simulink model "simulation"  (R2018b)
settings: Solver=FixedStepDiscrete  StartTime=0.0  StopTime=simtime  FixedStep=stepsize  RelTol=1e-3
undefined symbols (not defined in the file): activate_stop, activate_stop_vmax, ay_stop, Bat_param, deltav_ist, DiscIntNeverNeededParam, EG_wunsch, magnitude, mu_road_LF, mu_road_LR, mu_road_RF, mu_road_RR, par_ASR, par_MDT, par_TIR, par_VEH, select_delta_h, select_M_wheel, stepsize, t, temp_betriebsstrategie, temperature_LTrange, track_left, track_right
libraries: Library_ASK x36, simulink x18, dspstat3 x2, Library_Betriebsstrategie x2, vehicle_model x2, pacejka_trans x1
(part 6 of 6)

== system simulation/Vehicle/Betriebsstrategie/Momentenverteilung_und_Schaltstrategie1/Radmomentenaufteilung (Effizienz)/Torque shift damper/Optimierung_damped_AWD ==
  P_achs : Inport
  M_target : Inport  Port=2
  Enable : EnablePort
  Constant : Constant  Value=0.022
  Constant1 : Constant  Value=2
  Memory : Memory  InitialCondition=1
  Memory1 : Memory
  Memory2 : Memory  InitialCondition=1
  Minimierung : MATLAB Function  TreatAsAtomicUnit=on
  Product : Product
  Sign : Signum
  P_opt : Outport
  ind : Outport  Port=2
  wires:
  P_achs/1 -> Minimierung/1(P_achs)
  M_target/1 -> Product/1, Minimierung/4(M_target), Memory2/1
  Constant/1 -> Minimierung/2(difference)
  Memory2/1 -> Product/2
  Constant1/1 -> Minimierung/3(max_oscillation_sec)
  Minimierung/2(ind) -> ind/1, Memory/1
  Memory1/1 -> Minimierung/7(count_prev)
  Memory/1 -> Minimierung/6(ind_prev)
  Minimierung/3(count) -> Memory1/1
  Minimierung/1(P_opt) -> P_opt/1
  Product/1 -> Sign/1
  Sign/1 -> Minimierung/5(change)

== system simulation/Vehicle/Betriebsstrategie/Momentenverteilung_und_Schaltstrategie1/Radmomentenaufteilung (Effizienz)/Torque shift damper/Optimierung_eine_achs ==
  P_achs : Inport
  M_target : Inport  Port=2
  Akt_VA : Inport  Port=3
  Akt_HA : Inport  Port=4
  Enable : EnablePort
  Optimierung : MATLAB Function  TreatAsAtomicUnit=on
  "P_opt " : Outport
  "ind " : Outport  Port=2
  wires:
  Optimierung/1(P_opt) -> "P_opt "/1
  Optimierung/2(ind) -> "ind "/1
  M_target/1 -> Optimierung/2(M_target)
  P_achs/1 -> Optimierung/1(P_achs)
  Akt_VA/1 -> Optimierung/3(VA)
  Akt_HA/1 -> Optimierung/4(HA)

== system simulation/Vehicle/Betriebsstrategie/Momentenverteilung_und_Schaltstrategie1/Radmomentenaufteilung (Effizienz)/Momentenrückführung und Motormomentberechnung/Getriebewirkungsgradberechnung Hinterachse/Falls radnahe Maschine an HA1 ==
  M_HA : Inport
  Constant1 : Constant  Value=par_MDT.AUS.akt.az_HA
  Gain : Gain  Gain=0.5
  Switch : Switch  Criteria=u2 > Threshold
  M_HA_mot : Outport
  wires:
  Constant1/1 -> Switch/2
  M_HA/1 -> Switch/1, Gain/1
  Gain/1 -> Switch/3
  Switch/1 -> M_HA_mot/1

== system simulation/Vehicle/Betriebsstrategie/Momentenverteilung_und_Schaltstrategie1/Radmomentenaufteilung (Effizienz)/Momentenrückführung und Motormomentberechnung/Getriebewirkungsgradberechnung Hinterachse/Falls radnahe Maschine an HA2 ==
  M_HA : Inport
  Constant1 : Constant  Value=par_MDT.AUS.akt.az_HA
  Gain : Gain  Gain=2
  Switch : Switch  Criteria=u2 > Threshold
  M_HA_mot : Outport
  wires:
  Constant1/1 -> Switch/2
  M_HA/1 -> Switch/1, Gain/1
  Gain/1 -> Switch/3
  Switch/1 -> M_HA_mot/1

== system simulation/Vehicle/Betriebsstrategie/Momentenverteilung_und_Schaltstrategie1/Radmomentenaufteilung (Effizienz)/Momentenrückführung und Motormomentberechnung/Getriebewirkungsgradberechnung Vorderachse/Falls radnahe Maschine an VA ==
  M_VA : Inport
  Constant1 : Constant  Value=par_MDT.AUS.akt.az_VA
  Gain : Gain  Gain=0.5
  Switch : Switch  Criteria=u2 > Threshold
  M_VA_mot : Outport
  wires:
  Constant1/1 -> Switch/2
  M_VA/1 -> Switch/1, Gain/1
  Gain/1 -> Switch/3
  Switch/1 -> M_VA_mot/1

== system simulation/Vehicle/Betriebsstrategie/Momentenverteilung_und_Schaltstrategie1/Radmomentenaufteilung (Effizienz)/Momentenrückführung und Motormomentberechnung/Getriebewirkungsgradberechnung Vorderachse/Falls radnahe Maschine an VA1 ==
  M_VA : Inport
  Constant1 : Constant  Value=par_MDT.AUS.akt.az_VA
  Gain : Gain  Gain=2
  Switch : Switch  Criteria=u2 > Threshold
  M_VA_mot : Outport
  wires:
  Constant1/1 -> Switch/2
  M_VA/1 -> Switch/1, Gain/1
  Gain/1 -> Switch/3
  Switch/1 -> M_VA_mot/1

== matlab function simulation/Driver/Splines/Kennwerte ==
  data: psi_old input; psi_spline output; time input; a1 input; a0 input; v2 input; v1 input; v0 input; p3 input; p2 input; p1 input; p0 input; psi_real input; spl_a_glob output; spl_v_glob output; spl_p_glob output; spl_a_veh output; spl_v_veh output; p_err_long output; p_ist input; p_err_lat output
function [ psi_spline, spl_a_glob, spl_v_glob, spl_p_glob, spl_a_veh, spl_v_veh, p_err_long, p_err_lat]   = Kennwerte(psi_old, time, a1, a0, v2, v1, v0, p3, p2, p1, p0, psi_real, p_ist) 
%Splinekoeffizienten im Abstand von 0.01 s, deshalb wird Zeit mit 100 
%mulitpliziert,um alle 0.01 s auf nächsten Spline-Koeffizienten zuzugreifen
time = time * 100;
%t wird angelegt, damit extrapoliert werden kann, wenn die Zeit über die
%vorgesehene Zeit im Struct hinausreicht
t = time;
if time > length(a0)-2
    time = length(a0)-2;
end

si = int16(floor(time)+1); %Spline Index, Auswahl des Richtigen Splines 
ov = t-floor(time); %Overshoot, Zeit nach dem Beginn des Spline

%%Berechnung der Beschleunigung a, Geschwindigkeit v und Position p in globalen Koordianten
spl_a_glob =  a1(:,si).*(ov)   +a0(:,si);
spl_v_glob =  v2(:,si).*(ov).^2+v1(:,si).*(ov)   +v0(:,si);
spl_p_glob =  p3(:,si).*(ov).^3+p2(:,si).*(ov).^2+p1(:,si).*(ov)+p0(:,si);

%%Verhindert Springen des Gierwinkels bei niedrigen Geschwindigkeiten
if spl_v_glob(1) < 1e-5 && spl_v_glob(2) < 1e-5
     psi_spline = psi_old;
else
     psi_spline = atan2(spl_v_glob(2),spl_v_glob(1)); %Gierwinkel soll
end

psi = psi_spline; %Optional kann die tatsächliche Fahrzeugausrichtung verwendet werden
tm  = [cos(psi) sin(psi); -sin(psi) cos(psi)]; %Transformations-Matrix

spl_a_veh = tm * spl_a_glob; %Beschleunigung soll in Fahrzeugsollkoordinaten
spl_v_veh = tm * spl_v_glob; %Geschwindigkeit soll in Fahrzeugsollkoordinaten


p_veh = tm * (p_ist - spl_p_glob);
p_err_long = p_veh(1); %Lateraler Fehler in Fahrzeugsollkoordinaten
p_err_lat = p_veh(2); %Longitudinaler in Fahrzeugsollkoordinaten

end

== matlab function simulation/Vehicle/Antriebsstrang und Radmomentenverteilung/Batterie/MATLAB Function2 ==
  data: u input; y output
function y = fcn(u)
%Transponieren der Leistung -> für das Batteriemodell

y=reshape(u,[1,1,[]]);


end

== matlab function simulation/Vehicle/Betriebsstrategie/Momentenverteilung_und_Schaltstrategie1/Radmomentenaufteilung (Effizienz)/Momentenrückführung und Motormomentberechnung/Getriebewirkungsgradberechnung Vorderachse/MATLAB Function ==
  data: M_out input; M_in output; M_max input
function M_in = fcn(M_out, M_max)
M_in = 3/680 *((sqrt(M_max) * sqrt(27*M_max + 27200*M_out))/sqrt(3) - 3 * M_max)

== matlab function simulation/Driver/driver lateral/Pure Pursuit/MATLAB Function ==
  data: oldtime input; lad input; time input; v2 input; v1 input; v0 input; p3 input; p2 input; p1 input; p0 input; p_ist input; time_out output; dt output; err output; cp output
function [time_out, dt, err, cp]    = Carott(oldtime, lad, time,v2, v1, v0, p3, p2, p1, p0, p_ist)

t = oldtime; %Übernahme der Zeit aus letztem Zeitschritt

%Verhindert einen Zeitindex außerhalb der Matrixgröße
if oldtime > length(p0)-2
    oldtime = length(p0)-2;
elseif oldtime < 0
    oldtime = 0
end


si = int16(floor(oldtime)+1); %Spline Index, Auswahl des Richtigen Splines 
ov = t-floor(oldtime); %Overshoot, Zeit nach dem Beginn des Spline
cp =  p3(:,si).*(ov).^3+p2(:,si).*(ov).^2+p1(:,si).*(ov)+p0(:,si); %Berechnung des CP bei prognostizierter Zeit 


dist = norm(cp-p_ist); %Abstand Carrot-Point zum Fahrzeug
err = abs(1-dist/lad) %Normierung des Fehlers auf LAD
dt = 0; %Zeitdifferenz wird genullt

    v =  norm(v2(:,si).*(ov).^2+v1(:,si).*(ov)  +v0(:,si)); %FZG-Geschwindigkeit wird berechnet
    if v < 0.3 %Mindestgeschwindigkeit um CP bei Stillstand zu ermitteln 
        v = 0.3
    end
    dt = dt + (lad-dist)/v*100; %Zeitdifferenz wird aus Abstandsfehler und Geschwindigkeit ermittelt
    newtime = oldtime + dt; %Neuer Zeitpunkt, auf dem sich CP befindet, wird prognostiziert
    t = newtime; %Übernahme der prognostizierten Zeit
    
    %Verhindert einen Zeitindex außerhalb der Matrixgröße
    if newtime > length(p0)-2
        newtime = length(p0)-2;
    elseif newtime < 0
        newtime = 0
    end
    
    si = int16(floor(newtime)+1); %Spline Index, Auswahl des Richtigen Splines 
    ov = t-floor(newtime); %Overshoot, Zeit nach dem Beginn des Spline
    cp =  p3(:,si).*(ov).^3+p2(:,si).*(ov).^2+p1(:,si).*(ov)+p0(:,si); %Berechnung des CP bei neuer prognostizierter Zeit 
    dist = norm(cp-p_ist); %Abstand Carrot-Point zum Fahrzeug
    err = abs(1-dist/lad) %Normierung des Fehlers auf LAD

time_out = oldtime + dt; %Neuer Zeitpunkt, auf dem sich CP befindet, wird prognostiziert
end

== matlab function simulation/Vehicle/Betriebsstrategie/Momentenverteilung_und_Schaltstrategie1/Radmomentenaufteilung (Effizienz)/Momentenrückführung und Motormomentberechnung/Getriebewirkungsgradberechnung Hinterachse/MATLAB Function1 ==
  data: M_out input; M_in output; M_max input
function M_in = fcn(M_out, M_max)
M_in = 3/680 *((sqrt(M_max) * sqrt(27*M_max + 27200*M_out))/sqrt(3) - 3 * M_max)

== matlab function simulation/Vehicle/Antriebsstrang und Radmomentenverteilung/Batterie/MATLAB Function3 ==
  data: u input; y output
function y = fcn(u)
%Zusammenfassung der Verluste der LE auf eine Vektorspalte -> für das
%Batteriemodell


y=reshape(u,[[],1,1]);



end

== matlab function simulation/Vehicle/Antriebsstrang und Radmomentenverteilung/MATLAB Function2 ==
  data: u input; RIX output
function RIX = fcn(u)
%RIX = 1 für Antrieb an mindestens einem Rad, sonst -1
s = (sign(u) == 1);
if all(s) == 0
    RIX = -1;
else
    RIX = 1;
end
end

== matlab function simulation/Vehicle/Antriebsstrang und Radmomentenverteilung/MATLAB Function3 ==
  data: u input; RIX output
function RIX = fcn(u)
%RIX = 1 für Antrieb an mindestens einem Rad, sonst -1
s = (sign(u) == 1);
if all(s) == 0
    RIX = -1;
else
    RIX = 1;
end
end

== matlab function simulation/Vehicle/Betriebsstrategie/Momentenverteilung_und_Schaltstrategie1/Limitierungen gesamt (mit MVS Limits)/Aktuatoren und Delta TV/TV Moment pro Achse ==
  data: L1 input; Delta_T_f output; L2 input; L3 input; L4 input; L5 input; a_f input; a_r input; Delta_T_r output
function [Delta_T_f, Delta_T_r]  = fcn(L1, L2, L3, L4, L5, a_f, a_r)

%% Initialisierung
Delta_T_f=0;
Delta_T_r=0;

%% Zuweisung der maximalen TV Momente anhand der Antriebsstrangtopologie
if a_f == 3
    Delta_T_f=L5;
elseif a_f == 4
    Delta_T_f=L1;
elseif a_f == 5
    Delta_T_f=L2;
end

if a_r == 3
    Delta_T_r=L5;
elseif a_r == 4
    Delta_T_r=L1;
elseif a_r == 5
    Delta_T_r=L2;
end

%% Nomenklatur der Aktuatoren a_r und a_f
    % 1 = nur Elektromaschinen an der Achse
    % 2 = Offenes Differential an der Achse
    % 3 = Limited Slip Differential an der Achse
    % 4 = Elektrisches Überlagerungsgetriebe an der Achse
    % 5 = Mechanisches Überlagerungsgetriebe an der Achse

== matlab function simulation/Vehicle/Antriebsstrang und Radmomentenverteilung/MATLAB Function4 ==
  data: u input; RIX output
function RIX = fcn(u)
%RIX = 1 für Antrieb an mindestens einem Rad, sonst -1
s = (sign(u) == 1);
if all(s) == 0
    RIX = -1;
else
    RIX = 1;
end
end

== matlab function simulation/Vehicle/Antriebsstrang und Radmomentenverteilung/MATLAB Function5 ==
  data: u input; RIX output
function RIX = fcn(u)
%RIX = 1 für Antrieb an mindestens einem Rad, sonst -1
s = (sign(u) == 1);
if all(s) == 0
    RIX = -1;
else
    RIX = 1;
end
end

== matlab function simulation/Vehicle/Betriebsstrategie/Momentenverteilung_und_Schaltstrategie1/Limitierungen gesamt (mit MVS Limits)/Aktuatoren und Delta TV/Zuweisung Aktuatoren ==
  data: A1 input; A2 input; A3 input; A4 input; A5 input; a_f output; a_r output; A6 input; A7 input; A8 input; A9 input; A10 input
function [a_f, a_r]  = fcn(A1, A2, A3, A4, A5, A6, A7, A8, A9, A10)

%% Initialisierung
a_f=1;
a_r=1;

%% Zuweisung der Aktuatoren
% vorne
if A1 == 1
    a_f = 2;
elseif A2 == 1
    a_f = 3;
elseif A3 == 1
    a_f = 5;
elseif A4 == 1
    a_f = 4;
elseif A5 == 1
    a_f = 1;
end

% hinten
if A6 == 1
    a_r = 2;
elseif A7 == 1
    a_r = 3;
elseif A8 == 1
    a_r = 5;
elseif A9 == 1
    a_r = 4;
elseif A10 == 1
    a_r = 1;
end

%% Nomenklatur der Aktuatoren a_r und a_f
    % 1 = nur Elektromaschinen an der Achse
    % 2 = Offenes Differential an der Achse
    % 3 = Limited Slip Differential an der Achse
    % 4 = Elektrisches Überlagerungsgetriebe an der Achse
    % 5 = Mechanisches Überlagerungsgetriebe an der Achse

== matlab function simulation/Vehicle/Antriebsstrang und Radmomentenverteilung/MATLAB Function ==
  data: u input; RIX output
function RIX = fcn(u)
%RIX = 1 für Antrieb an mindestens einem Rad, sonst -1
s = (sign(u) == 1);
if all(s) == 0
    RIX = -1;
else
    RIX = 1;
end
end

== matlab function simulation/Vehicle/Antriebsstrang und Radmomentenverteilung/MATLAB Function1 ==
  data: u input; RIX output
function RIX = fcn(u)
%RIX = 1 für Antrieb an mindestens einem Rad, sonst -1
s = (sign(u) == 1);
if all(s) == 0
    RIX = -1;
else
    RIX = 1;
end
end

== matlab function simulation/Vehicle/Betriebsstrategie/Momentenverteilung_und_Schaltstrategie1/Limitierungen gesamt (mit MVS Limits)/Limits Zusammenführung ==
  data: FxlimRF input; FxlimLF input; FxlimRR input; Fx_LF_ub output; Fx_LF_lb output; Fx_RF_ub output; Fx_RF_lb output; Fx_LR_ub output; Fx_LR_lb output; Fx_RR_ub output; Fx_RR_lb output; FxlimLR input; M_RF_ub input; M_RF_lb input; M_LF_ub input; M_LF_lb input; M_RR_ub input; M_RR_lb input; M_LR_ub input; M_LR_lb input; M_F_lb input; M_F_ub input; M_R_lb input; M_R_ub input; DELTA_T_f input; DELTA_T_r input; a_f input; a_r input; r input
function [Fx_LF_ub, Fx_LF_lb, Fx_RF_ub, Fx_RF_lb, Fx_LR_ub, Fx_LR_lb, Fx_RR_ub, Fx_RR_lb] = fcn(FxlimRF, FxlimLF, FxlimRR, FxlimLR, M_RF_ub, M_RF_lb, M_LF_ub, M_LF_lb, M_RR_ub, M_RR_lb, M_LR_ub, M_LR_lb, M_F_lb, M_F_ub, M_R_lb, M_R_ub,DELTA_T_f, DELTA_T_r,a_f, a_r, r)

% Reifenverhalten beim Antreiben und Bremsen gleich
Fx_LF_ub = FxlimLF;
Fx_RF_ub = FxlimRF;
Fx_LF_lb = (-1*FxlimLF);
Fx_RF_lb = (-1*FxlimRF);

Fx_LR_ub = FxlimLR;
Fx_RR_ub = FxlimRR;
Fx_LR_lb = (-1*FxlimLR);
Fx_RR_lb = (-1*FxlimRR);

% Notwendig, da die Rekuperationskennfelder aus dem Pesche Tool positive
% Momente ausgeben
M_RF_lb=(-1)*M_RF_lb;
M_LF_lb=(-1)*M_LF_lb;
M_RR_lb=(-1)*M_RR_lb;
M_LR_lb=(-1)*M_LR_lb;
M_F_lb=(-1)*M_F_lb;
M_R_lb=(-1)*M_R_lb;
    
%% Nomenklatur der Aktuatoren a_r und a_f
    % 1 = nur Elektromaschinen an der Achse
    % 2 = Offenes Differential an der Achse
    % 3 = Limited Slip Differential an der Achse
    % 4 = Elektrisches Überlagerungsgetriebe an der Achse
    % 5 = Mechanisches Überlagerungsgetriebe an der Achse
 
    
%% Nur Elektromotoren: Limit ist Minimum/Maximum aus Reifenlimit und Limit der EM
if a_f == 1
    Fx_LF_ub = min(FxlimLF,(M_LF_ub/r));
    Fx_RF_ub = min(FxlimRF,(M_RF_ub/r));
    Fx_LF_lb = max((-1*FxlimLF),(M_LF_lb/r));
    Fx_RF_lb = max((-1*FxlimRF),(M_RF_lb/r));
end

if a_r == 1
    Fx_LR_ub = min(FxlimLR,(M_LR_ub/r));
    Fx_RR_ub = min(FxlimRR,(M_RR_ub/r));
    Fx_LR_lb = max((-1*FxlimLR),(M_LR_lb/r));
    Fx_RR_lb = max((-1*FxlimRR),(M_RR_lb/r));
end

%% Offenes Differential: Limit ist Minimum/Maximum aus Reifenlimit und genau der Hälfte des max. Moments der achszentralen EM
if a_f == 2
    Fx_LF_ub = min(FxlimLF,(0.5*M_F_ub/r));
    Fx_RF_ub = min(FxlimRF,(0.5*M_F_ub/r));
    Fx_LF_lb = max((-1*FxlimLF),(0.5*M_F_lb/r));
    Fx_RF_lb = max((-1*FxlimRF),(0.5*M_F_lb/r));
end

if a_r == 2
    Fx_LR_ub = min(FxlimLR,(0.5*M_R_ub/r));
    Fx_RR_ub = min(FxlimRR,(0.5*M_R_ub/r));
    Fx_LR_lb = max((-1*FxlimLR),(0.5*M_R_lb/r));
    Fx_RR_lb = max((-1*FxlimRR),(0.5*M_R_lb/r));
end

%% Limited Slip Differential %% Elektrisches Überlagerungsgetriebe %% Mechanisches Überlagerungsgetriebe:
if a_f >= 3 
    Fx_LF_ub = min(FxlimLF,(0.5*M_F_ub/r + 0.5*DELTA_T_f/r));
    Fx_RF_ub = min(FxlimRF,(0.5*M_F_ub/r + 0.5*DELTA_T_f/r));
    Fx_LF_lb = max((-1*FxlimLF),(0.5*M_F_lb/r - 0.5*DELTA_T_f/r));
    Fx_RF_lb = max((-1*FxlimRF),(0.5*M_F_lb/r - 0.5*DELTA_T_f/r));
end

if a_r >= 3
    Fx_LR_ub = min(FxlimLR,(0.5*M_R_ub/r + 0.5*DELTA_T_r/r));
    Fx_RR_ub = min(FxlimRR,(0.5*M_R_ub/r + 0.5*DELTA_T_r/r));
    Fx_LR_lb = max((-1*FxlimLR),(0.5*M_R_lb/r - 0.5*DELTA_T_r/r));
    Fx_RR_lb = max((-1*FxlimRR),(0.5*M_R_lb/r - 0.5*DELTA_T_r/r));
end


%% kein Antrieb an der achse
if a_f >= 4
    Fx_LF_ub = min(FxlimLF,(0.5*M_F_ub/r + 0.5*DELTA_T_f/r));
    Fx_RF_ub = min(FxlimRF,(0.5*M_F_ub/r + 0.5*DELTA_T_f/r));
    Fx_LF_lb = max((-1*FxlimLF),(0.5*M_F_lb/r - 0.5*DELTA_T_f/r));
    Fx_RF_lb = max((-1*FxlimRF),(0.5*M_F_lb/r - 0.5*DELTA_T_f/r));
end

if a_r >= 4
    Fx_LR_ub = min(FxlimLR,(0.5*M_R_ub/r + 0.5*DELTA_T_r/r));
    Fx_RR_ub = min(FxlimRR,(0.5*M_R_ub/r + 0.5*DELTA_T_r/r));
    Fx_LR_lb = max((-1*FxlimLR),(0.5*M_R_lb/r - 0.5*DELTA_T_r/r));
    Fx_RR_lb = max((-1*FxlimRR),(0.5*M_R_lb/r - 0.5*DELTA_T_r/r));
end

%% Torque Splitter
if a_f == 5
    Fx_LF_ub = min(FxlimLF,(M_F_ub/r));
    Fx_RF_ub = min(FxlimRF,(M_F_ub/r));
    Fx_LF_lb = max((-1*FxlimLF),(M_F_lb/r - DELTA_T_f/r));
    Fx_RF_lb = max((-1*FxlimRF),(M_F_lb/r - DELTA_T_f/r));
end

if a_r == 5
    Fx_LR_ub = min(FxlimLR,(M_R_ub/r));
    Fx_RR_ub = min(FxlimRR,(M_R_ub/r));
    Fx_LR_lb = max((-1*FxlimLR),(M_R_lb/r - DELTA_T_r/r));
    Fx_RR_lb = max((-1*FxlimRR),(M_R_lb/r - DELTA_T_r/r));
end

== matlab function simulation/Vehicle/Betriebsstrategie/Momentenverteilung_und_Schaltstrategie1/Radmomentenaufteilung (Effizienz)/Torque shift damper/Optimierung_eine_achs/Optimierung ==
  data: P_achs input; P_opt output; ind output; M_target input; VA input; HA input
function [P_opt, ind]= fcn(P_achs, M_target, VA, HA)

[n_gears, leng] = size(P_achs);

if HA == 1
    if M_target>0
        [P_opt, ind] = min(P_achs(:,1));
    else
        [P_opt, ind] = max(P_achs(:,1));
    end
else
    if M_target>0
        [P_opt, ind] = min(P_achs(:,leng));
    else
        [P_opt, ind] = max(P_achs(:,leng));
    end
    ind = ind+100*n_gears
end

end

== matlab function simulation/Vehicle/Betriebsstrategie/Momentenverteilung_und_Schaltstrategie1/Radmomentenaufteilung (Standardfahrmanöver)/Limits berücksichtigen ==
  data: Fx_RF output; Fx_LF output; Fx_RR output; Fx_LF_ub input; Fx_LF_lb input; Fx_RF_ub input; Fx_RF_lb input; Fx_LR_ub input; Fx_LR_lb input; Fx_RR_ub input; Fx_RR_lb input; a_f input; a_r input; Fx_LR output; X_FL input; X_FR input; X_RL input; X_RR input
function [Fx_RF, Fx_LF, Fx_RR, Fx_LR] = fcn(Fx_LF_ub, Fx_LF_lb, Fx_RF_ub, Fx_RF_lb, Fx_LR_ub, Fx_LR_lb, Fx_RR_ub, Fx_RR_lb,a_f, a_r, X_FL, X_FR, X_RL, X_RR)

%% Initialisierung
Fx_RF = X_FR;
Fx_LF = X_FL;
Fx_RR = X_RR;
Fx_LR = X_RL;
    
%% Nomenklatur der Aktuatoren a_r und a_f
    % 1 = nur Elektromaschinen an der Achse
    % 2 = Offenes Differential an der Achse
    % 3 = Limited Slip Differential an der Achse
    % 4 = Elektrisches Überlagerungsgetriebe an der Achse
    % 5 = Mechanisches Überlagerungsgetriebe an der Achse
 
%% Algorithmus

    F_f= Fx_RF+Fx_LF;
    F_r= Fx_RR+Fx_LR;
  
  % Nur Elektromotoren:
  % Es werden radindividuell die Grenzen eingehalten. Die Differenzkräfte
  % werden zur späteren Verwendung gespeichert.
if a_f ==1
    if Fx_LF > Fx_LF_ub
        dFx_LF = Fx_LF-Fx_LF_ub;
        Fx_LF = Fx_LF_ub;
    end
    if Fx_RF > Fx_RF_ub
        dFx_RF = Fx_RF-Fx_RF_ub;
        Fx_RF = Fx_RF_ub;
    end
    if Fx_LF < Fx_LF_lb
        dFx_LF = Fx_LF-Fx_LF_lb;
        Fx_LF = Fx_LF_lb;
    end
    if Fx_RF < Fx_RF_lb
        dFx_RF = Fx_RF-Fx_RF_lb;
        Fx_RF = Fx_RF_lb;
    end
end

if a_r ==1
    if Fx_LR > Fx_LR_ub
        dFx_LR = Fx_LR-Fx_LR_ub;
        Fx_LR = Fx_LR_ub;
    end
    if Fx_RR > Fx_RR_ub
        dFx_RR = Fx_RR-Fx_RR_ub;
        Fx_RR = Fx_RR_ub;
    end
    if Fx_LR < Fx_LR_lb
        dFx_LR = Fx_LR-Fx_LR_lb;
        Fx_LR = Fx_LR_lb;
    end
    if Fx_RR < Fx_RR_lb
        dFx_RR = Fx_RR-Fx_RR_lb;
        Fx_RR = Fx_RR_lb;
    end
end

  % Offenes Differential:
  % ALSO keine TV Funktion der Achse.
  % Jedes Rad erhält die Hälfte der Gesamtachskraft.
  % Anschließend wird diese Kraft auf das Minimum der einzelnen Limits
  % gedeckelt.

  %Berücksichtigung bereits in Lagrange-Block
  
if a_f ==2
    Fx_LF = F_f/2;
    Fx_RF = F_f/2;
    if Fx_LF > Fx_LF_ub || Fx_RF > Fx_RF_ub
        Fx_LF = min(Fx_LF_ub,Fx_RF_ub);
        Fx_RF = Fx_LF;
    end
    if Fx_LF < Fx_LF_lb || Fx_RF < Fx_RF_lb
        Fx_LF = max(Fx_LF_lb,Fx_RF_lb);
        Fx_RF = Fx_LF;
    end
end

if a_r ==2
    Fx_LR = F_r/2;
    Fx_RR = F_r/2;
    if Fx_LR > Fx_LR_ub || Fx_RR > Fx_RR_ub
        Fx_LR = min(Fx_LR_ub,Fx_RR_ub);
        Fx_RR = Fx_LR;
    end
    if Fx_LR < Fx_LR_lb || Fx_RR < Fx_RR_lb
        Fx_LR = max(Fx_LR_lb,Fx_RR_lb);
        Fx_RR = Fx_LR;
    end
end
    
%% Limited Slip Differential %% Elektrisches Überlagerungsgetriebe %% Mechanisches Überlagerungsgetriebe
if a_f >=3
    if Fx_LF > Fx_LF_ub
        dFx_LF = Fx_LF-Fx_LF_ub;
        Fx_LF = Fx_LF_ub;
    end
    if Fx_RF > Fx_RF_ub
        dFx_RF = Fx_RF-Fx_RF_ub;
        Fx_RF = Fx_RF_ub;
    end
    if Fx_LF < Fx_LF_lb
        dFx_LF = Fx_LF-Fx_LF_lb;
        Fx_LF = Fx_LF_lb;
    end
    if Fx_RF < Fx_RF_lb
        dFx_RF = Fx_RF-Fx_RF_lb;
        Fx_RF = Fx_RF_lb;
    end
end

if a_r >=3
    if Fx_LR > Fx_LR_ub
        dFx_LR = Fx_LR-Fx_LR_ub;
        Fx_LR = Fx_LR_ub;
    end
    if Fx_RR > Fx_RR_ub
        dFx_RR = Fx_RR-Fx_RR_ub;
        Fx_RR = Fx_RR_ub;
    end
    if Fx_LR < Fx_LR_lb
        dFx_LR = Fx_LR-Fx_LR_lb;
        Fx_LR = Fx_LR_lb;
    end
    if Fx_RR < Fx_RR_lb
        dFx_RR = Fx_RR-Fx_RR_lb;
        Fx_RR = Fx_RR_lb;
    end
end
    
%% Korrektur des TV Moments %% Korrektur des Gesamtmoments

== matlab function simulation/Vehicle/Betriebsstrategie/Momentenverteilung_und_Schaltstrategie1/Radmomentenaufteilung (Effizienz)/Torque shift damper/Optimierung_damped_AWD/Minimierung ==
  data: P_achs input; P_opt output; ind output; count output; difference input; max_oscillation_sec input; M_target input; change input; ind_prev input; count_prev input
function [P_opt, ind, count]= fcn(P_achs, difference, max_oscillation_sec, M_target, change, ind_prev, count_prev)

[leng, x] = size(P_achs);
if M_target>0
    [P_opt, ind] = min(P_achs(:));

    if (P_opt < (1-difference)*P_achs(ind_prev) && count_prev > (leng*2000/max_oscillation_sec)) || change == -1 || isnan(P_achs(ind_prev)) == 1
        count = 0
    else
        ind = ind_prev;
        P_opt = P_achs(ind_prev);
        count = count_prev+1;
    end

else
    [P_opt, ind] = max(P_achs(:));
    
    if (P_opt > (1+difference)*P_achs(ind_prev) && count_prev > (leng*2000/max_oscillation_sec)) || change == -1 || isnan(P_achs(ind_prev)) == 1
        count = 0
    else
        ind = ind_prev;
        P_opt = P_achs(ind_prev);
        count = count_prev+1;
    end
end

end

== matlab function simulation/Vehicle/Betriebsstrategie/Momentenverteilung_und_Schaltstrategie1/Radmomentenaufteilung (Standardfahrmanöver)/Optimierung mit Lagrange Multiplikator Methode ==
  data: a_f input; a_r input; X_req input; Z_FL input; Z_FR input; Z_RL input; Z_RR input; Mz input; tF input; tR input; lf input; lr input; delta input; X_FL output; X_FR output; X_RL output; X_RR output; X_FL1 input; X_FR1 input; X_RL1 input; X_RR1 input
function [X_FL, X_FR, X_RL, X_RR] = fcn(a_f, a_r, X_req, Z_FL, Z_FR, Z_RL, Z_RR, Mz, tF, tR, lf, lr, delta, X_FL1, X_FR1, X_RL1, X_RR1)

%% Auswahl der Antriebsstrantopologie
a=1;
b=1;

if a_f ==2
    a=0;
end
if a_r ==2
    b=0;
end

if a_f ==2 && a_r==2
    a=1;
    b=1;
end

% TV vorne und hinten möglich a=1 und b=1
% TV nur vorne möglich a=1
% TV nur hinten möglich b=1
% kein TV möglich a=1 und b=1 und anschließend gleichmäßig aufteilen

%% Matrix für die Randbedingungen ( Gesamtmoment und TV Moment)
% B0 = [cos(delta) cos(delta) 1 1; a*((-tF/2)*cos(delta)+lf*sin(delta)) a*((tF/2)*cos(delta)+lf*sin(delta)) b*(-tR/2) b*(tR/2)];
% Die Berücksichtigung der Lenkwinkel für die Formel des Gesamtmoments und des Giermomenmts ist exakt, wird
% aber hier erstmal auskommentiert, da ein instabiler Fahrerregler
% vorliegt. Sobald der Fahrerregler komplett stabil ist, kann die obere
% Matrix für B0 verwendet werden.
B0 = [1 1 1 1; a*(-tF/2) a*(tF/2) b*(-tR/2) b*(tR/2)];
y0 = [X_req; Mz];

%% Algorithmus
    %% Initialbedingungen
i=0;    
B=B0;
y=y0;
     
    %% Verhindern abgehobener Räder
if Z_FL < 1
    Z_FL = 1;
    x_FL_max = 0;
end

if Z_FR < 1
    Z_FR = 1;
    x_FR_max = 0;
end

if Z_RL < 1
    Z_RL = 1;
    x_RL_max = 0;
end

if Z_RR < 1
    Z_RR = 1;
    x_RR_max = 0;
end

%% Matrizen für die Mimimierung
W1 = [1/Z_FL 0 0 0; 0 1/Z_FR 0 0; 0 0 1/Z_RL 0; 0 0 0 1/Z_RR];
W2 = 0.01 * eye(4);
%Wquad = W1^2 + W2^2;
Wquad = W1 + W2^2;
X_alt = [X_FL1; X_FR1; X_RL1; X_RR1];

%% Minimierungsargument
% min ||W1*x||^2 + ||W2*(x-x0)||^2
%   ||W1*x||^2 + ||W2*(x-x0)||^2 = xt*W1^2*x + (x-x0)t*W2^2*(x-x0)
%   = xt*(W1^2+W2^2)*x - 2*x*W2^2*x0 + x0*W2^2*x0
%   = xt*W^2*x - 2*x*W2^2*x0 + Konstante
%   mit W^2 = W1^2 + W2^2

%% Berechnung von Xij
G = (Wquad^(-1))*(B')*(B*(Wquad^(-1))*(B'))^(-1);
X = G*y + (eye(4)-G*B)*(Wquad^(-1))*(W2^2)*X_alt;


%% Ausgabewerte berechnen
X_FL = X(1);
X_FR = X(2);
X_RL = X(3);
X_RR = X(4);

%% Limits berücksichtigen
if a==0
    X_F = X_FL + X_FR;
    X_FL = X_F/2;
    X_FR = X_F/2;
end

if b==0
    X_R = X_RL + X_RR;
    X_RL = X_R/2;
    X_RR = X_R/2;
end

if a_f ==2 && a_r==2
    X_F = X_FL + X_FR;
    X_FL = X_F/2;
    X_FR = X_F/2;
    X_R = X_RL + X_RR;
    X_RL = X_R/2;
    X_RR = X_R/2;
end

== matlab function simulation/Vehicle/Betriebsstrategie/Momentenverteilung_und_Schaltstrategie1/Radmomentenaufteilung (Standardfahrmanöver)/Schaltstrategie/Getriebe- wirkungs- grade ==
  data: eta_LF output; eta_RF output; eta_LR output; eta_RR output; eta_F output; eta_R output; idx_LF input; idx_RF input; idx_LR input; idx_RR input; idx_F input; idx_R input; ETA_F input; ETA_R input
function [eta_LF, eta_RF, eta_LR, eta_RR, eta_F, eta_R] = fcn(idx_LF, idx_RF, idx_LR, idx_RR, idx_F, idx_R, ETA_F, ETA_R)

eta_LF=ETA_F(idx_LF);
eta_RF=ETA_F(idx_RF);
eta_LR=ETA_R(idx_LR);
eta_RR=ETA_R(idx_RR);
eta_F=ETA_F(idx_F);
eta_R=ETA_R(idx_R);

% Der Wirkungsgrad des Getriebes im eingelegten Gang wird weitergegeben.
% Frederik benötigt diesen im Antriebsstrangmodell.

== matlab function simulation/Vehicle/Betriebsstrategie/Momentenverteilung_und_Schaltstrategie1/Radmomentenaufteilung (Standardfahrmanöver)/Schaltstrategie/Radmoment zu Motormoment ==
  data: i_LF input; i_RF input; i_LR input; i_RR input; i_F input; i_R input; M_LF input; m_LF output; M_RF input; M_LR input; M_RR input; m_RF output; m_LR output; m_RR output; m_F output; m_R output
function [m_LF, m_RF, m_LR, m_RR, m_F, m_R] = fcn(i_LF, i_RF, i_LR, i_RR, i_F, i_R, M_LF, M_RF, M_LR, M_RR)

%% Motormoment Achszentraler Aufbau
m_F=(M_LF+M_RF)/i_F;
m_R=(M_LR+M_RR)/i_R;

%% Motormoment Radindividueller Aufbau
m_LF=M_LF/i_LF;
m_RF=M_RF/i_RF;
m_LR=M_LR/i_LR;
m_RR=M_RR/i_RR;

== matlab function simulation/Vehicle/Betriebsstrategie/Momentenverteilung_und_Schaltstrategie1/Radmomentenaufteilung (Standardfahrmanöver)/Schaltstrategie/Schaltlogik ==
  data: delta_n_LF input; delta_n_RF input; delta_n_LR input; delta_n_RR input; delta_n_F input; delta_n_R input; delta_m_LF input; delta_m_RF input; delta_m_LR input; delta_m_RR input; delta_m_F input; delta_m_R input; idx_LF_eff input; idx_RF_eff input; idx_LR_eff input; idx_RR_eff input; idx_F_eff input; idx_R_eff input; i_LF output; i_RF output; i_LR output; i_RR output; i_F output; iv_LF input; iv_RF input; iv_LR input; iv_RR input; iv_F input; iv_R input; i_R output; idx_LF output; idx_RF output; idx_LR output; idx_RR output; idx_F output; idx_R output; idx_LF_alt input; idx_RF_alt input; idx_LR_alt input; idx_RR_alt input; idx_F_alt input; idx_R_alt input
function [i_LF, i_RF, i_LR, i_RR, i_F, i_R, idx_LF, idx_RF, idx_LR, idx_RR, idx_F, idx_R] = fcn(delta_n_LF, delta_n_RF, delta_n_LR, delta_n_RR, delta_n_F, delta_n_R, delta_m_LF, delta_m_RF, delta_m_LR, delta_m_RR, delta_m_F, delta_m_R, idx_LF_eff, idx_RF_eff, idx_LR_eff, idx_RR_eff, idx_F_eff, idx_R_eff, iv_LF, iv_RF, iv_LR, iv_RR, iv_F, iv_R, idx_LF_alt, idx_RF_alt, idx_LR_alt, idx_RR_alt, idx_F_alt, idx_R_alt)

%% Anzahl der möglichen Gänge
[A,max_LF]=size(iv_LF);
[A,max_RF]=size(iv_RF);
[A,max_LR]=size(iv_LR);
[A,max_RR]=size(iv_RR);
[A,max_F]=size(iv_F);
[A,max_R]=size(iv_R);

flag_LF=0;
flag_RF=0;
flag_LR=0;
flag_RR=0;
flag_F=0;
flag_R=0;


%% LF
idx_LF=idx_LF_alt;

if delta_n_LF<100 && idx_LF_alt<max_LF
    idx_LF=idx_LF_alt+1;
    flag_LF=1;
end

% if delta_m_LF<1 && idx_LF_alt>1 && flag_LF==0
%     idx_LF=idx_LF_alt-1;
%     flag_LF=1;
% end
    
if flag_LF==0
    idx_LF=idx_LF_eff;
end

i_LF=iv_LF(idx_LF);

%% RF
idx_RF=idx_RF_alt;

if delta_n_RF<100 && idx_RF_alt<max_RF
    idx_RF=idx_RF_alt+1;
    flag_RF=1;
end

% if delta_m_RF<1 && idx_RF_alt>1 && flag_RF==0
%     idx_RF=idx_RF_alt-1;
%     flag_RF=1;
% end
    
if flag_RF==0
    idx_RF=idx_RF_eff;
end

i_RF=iv_RF(idx_RF);

%% LR
idx_LR=idx_LR_alt;

if delta_n_LR<100 && idx_LR_alt<max_LR
    idx_LR=idx_LR_alt+1;
    flag_LR=1;
end

% if delta_m_LR<1 && idx_LR_alt>1 && flag_LR==0
%     idx_LR=idx_LR_alt-1;
%     flag_LR=1;
% end
    
if flag_LR==0
    idx_LR=idx_LR_eff;
end

i_LR=iv_LR(idx_LR);

%% RR
idx_RR=idx_RR_alt;

if delta_n_RR<100 && idx_RR_alt<max_RR
    idx_RR=idx_RR_alt+1;
    flag_RR=1;
end

% if delta_m_RR<1 && idx_RR_alt>1 && flag_RR==0
%     idx_RR=idx_RR_alt-1;
%     flag_RR=1;
% end
    
if flag_RR==0
    idx_RR=idx_RR_eff;
end

i_RR=iv_RR(idx_RR);

%% F
idx_F=idx_F_alt;

if delta_n_F<100 && idx_F_alt<max_F
    idx_F=idx_F_alt+1;
    flag_F=1;
end

% if delta_m_F<1 && idx_F_alt>1 && flag_F==0
%     idx_F=idx_F_alt-1;
%     flag_F=1;
% end
    
if flag_F==0
    idx_F=idx_F_eff;
end

i_F=iv_F(idx_F);

%% R
idx_R=idx_R_alt;

if delta_n_R<100 && idx_R_alt<max_R
    idx_R=idx_R_alt+1;
    flag_R=1;
end

% if delta_m_R<1 && idx_R_alt>1 && flag_R==0
%     idx_R=idx_R_alt-1;
%     flag_R=1;
% end
    
if flag_R==0
    idx_R=idx_R_eff;
end

i_R=iv_R(idx_R);

== matlab function simulation/Vehicle/Betriebsstrategie/Momentenverteilung_und_Schaltstrategie1/Radmomentenaufteilung (Standardfahrmanöver)/Schaltstrategie/effizientester Gang ==
  data: eta_LF input; eta_RF input; eta_LR input; eta_RR input; eta_F input; eta_R input; idx_LF_eff output; idx_RF_eff output; idx_LR_eff output; idx_RR_eff output; idx_F_eff output; idx_R_eff output; eta_trans_F input; eta_trans_R input
function [idx_LF_eff, idx_RF_eff, idx_LR_eff, idx_RR_eff, idx_F_eff, idx_R_eff] = fcn(eta_LF, eta_RF, eta_LR, eta_RR, eta_F, eta_R, eta_trans_F, eta_trans_R)

%% effizientester Gang Achszentraler Aufbau
[A,B]=max(eta_F .* eta_trans_F);
idx_F_eff=B;

[A,B]=max(eta_R .* eta_trans_R);
idx_R_eff=B;

%% effizientester Gang Radindividueller Aufbau
[A,B]=max(eta_LF .* eta_trans_F);
idx_LF_eff=B;

[A,B]=max(eta_RF .* eta_trans_F);
idx_RF_eff=B;

[A,B]=max(eta_LR .* eta_trans_R);
idx_LR_eff=B;

[A,B]=max(eta_RR .* eta_trans_R);
idx_RR_eff=B;

== matlab function simulation/Vehicle/Betriebsstrategie/Momentenverteilung_und_Schaltstrategie1/Radmomentenaufteilung (Standardfahrmanöver)/Schaltstrategie/n und Motordrehmoment als Vektor (wegen ALLEN Übersetzungen) ==
  data: omega_LF input; n_LF output; m_LF output; omega_RF input; omega_LR input; omega_RR input; M_LF input; M_RF input; M_LR input; M_RR input; i_LF input; i_RF input; i_LR input; i_RR input; i_F input; i_R input; n_RF output; m_RF output; n_LR output; m_LR output; n_RR output; m_RR output; n_F output; m_F output; n_R output; m_R output
function [n_LF,m_LF, n_RF,m_RF, n_LR,m_LR, n_RR,m_RR, n_F,m_F, n_R,m_R] = fcn(omega_LF, omega_RF, omega_LR, omega_RR, M_LF, M_RF, M_LR, M_RR, i_LF, i_RF, i_LR, i_RR, i_F, i_R)

%% Drehzahlen und Momente als Vektoren
% Die Menge an möglichen Übersetzungen liegt als Vektor vor.
% Durch Vektoropertaionen werden Drehzahlen und Momente ebenfalls als
% Vektoren dargestellt. Diese werden im Wirkungsgradkennfeld zu einem
% Vektor an Wirkungsgraden. Von diesen wird der beste ausgewählt.

%% Raddrehzahlen Achszentraler Aufbau
n_F = (omega_LF+omega_RF)*0.5.*i_F;
n_R = (omega_LR+omega_RR)*0.5.*i_R;

%% Raddrehzahlen Radindividueller Aufbau
n_LF = omega_LF.*i_LF;
n_RF = omega_RF.*i_RF;
n_LR = omega_LR.*i_LR;
n_RR = omega_RR.*i_RR;

%% Motormoment Achszentraler Aufbau
m_F=(M_LF+M_RF)./i_F;
m_R=(M_LR+M_RR)./i_R;

%% Motormoment Radindividueller Aufbau
m_LF=M_LF./i_LF;
m_RF=M_RF./i_RF;
m_LR=M_LR./i_LR;
m_RR=M_RR./i_RR;

== matlab function simulation/Vehicle/Betriebsstrategie/Momentenverteilung_und_Schaltstrategie1/Radmomentenaufteilung (Standardfahrmanöver)/Schaltstrategie/omega zu n ==
  data: omega_LF input; n_LF output; omega_RF input; omega_LR input; omega_RR input; i_LF input; i_RF input; i_LR input; i_RR input; i_F input; i_R input; n_RF output; n_LR output; n_RR output; n_F output; n_R output
function [n_LF, n_RF, n_LR, n_RR, n_F, n_R] = fcn(omega_LF, omega_RF, omega_LR, omega_RR, i_LF, i_RF, i_LR, i_RR, i_F, i_R)

%% Raddrehzahlen Achszentraler Aufbau
n_F = (omega_LF+omega_RF)*0.5*i_F;
n_R = (omega_LR+omega_RR)*0.5*i_R;

%% Raddrehzahlen Radindividueller Aufbau
n_LF = omega_LF*i_LF;
n_RF = omega_RF*i_RF;
n_LR = omega_LR*i_LR;
n_RR = omega_RR*i_RR;
